simulink model "cruise_control_sim"  (R2013a)
settings: Solver=ode1  StartTime=0.0  StopTime=50  FixedStep=0.1  RelTol=1e-3
PreLoadFcn:
  | load('cruise_control_sim.mat')
undefined symbols (not defined in the file): EngineRPM, EngineTRQ, FinalRatio, GearRatio, Kdrag, Ki, Kp, Mass, sigbuilder_block, WheelRadius
libraries: simulink x1
settings Model: Creator=luca  LastModifiedBy=luca

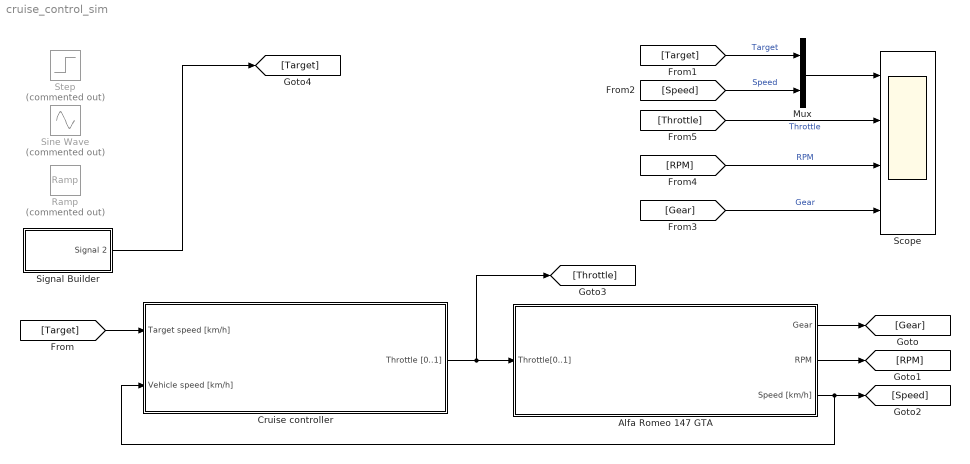
== system cruise_control_sim ==
  Alfa Romeo 147 GTA : Subsystem
  Cruise controller : Subsystem
  Mux : Mux  Inputs=2
  Ramp : simulink/Sources/Ramp  Commented=on  slope=6  start=0  X0=0
  Scope : Scope  NumInputPorts=4
      settings: ShowLegends=on  YMin=-5~-5~-5~-5  YMax=5~5~5~5
  Signal Builder : Subsystem  Tag=STV Subsys  LoadFcn=sigbuilder_block('load');  StartFcn=sigbuilder_block('start');  StopFcn=sigbuilder_block('stop');  ClipboardFcn=sigbuilder_block('clipboard');  mask(Sigbuilder block){}
      mask help: Simulink:masks:SigbuilderBlock_MD
      mask init:
      | if ~strcmp(get_param(bdroot(gcbh),'SimulationStatus'),'stopped') tuvar = sigbuilder_block('maskInit'); end
      settings: CopyFcn=sigbuilder_block('copy');  DeleteFcn=sigbuilder_block('delete');  ModelCloseFcn=sigbuilder_block('modelClose');  PreSaveFcn=sigbuilder_block('preSave');  PauseFcn=sigbuilder_block('pause');  ContinueFcn=sigbuilder_block('continue');  NameChangeFcn=sigbuilder_block('namechange');  OpenFcn=sigbuilder_block('open',[0 25.6 819.2 554.4 ]);  CloseFcn=sigbuilder_block('close');
      mask Display: plot(0, 0, 100, 100,[2, 2, 32, 32, 2], [68, 8, 8, 68, 68],[32, 2], [38, 38], [32, 19, 2],[53, 60, 44], [32, 17, 17, 2],[16, 16, 31, 31]);txt = getActiveGroup(gcbh);text(2, 100, txt,'verticalAlignment', 'top');
  Sine Wave : Sin  Commented=on  Amplitude=20  Bias=100  Frequency=0.2  SampleTime=0
  Step : Step  Commented=on  After=100  SampleTime=0
  wires:
  Cruise controller/1(Throttle [0..1]) -> Alfa Romeo 147 GTA/1(Throttle[0..1]), [Throttle]
  Alfa Romeo 147 GTA/3(Speed [km/h]) -> [Speed], Cruise controller/2(Vehicle speed [km/h])
  [Target] -> Cruise controller/1(Target speed [km/h])
  Alfa Romeo 147 GTA/1(Gear) -> [Gear]
  Alfa Romeo 147 GTA/2(RPM) -> [RPM]
  [Gear] -> Scope/4  "Gear"
  [RPM] -> Scope/3  "RPM"
  [Throttle] -> Scope/2  "Throttle"
  [Target] -> Mux/1  "Target"
  [Speed] -> Mux/2  "Speed"
  Mux/1 -> Scope/1
  Signal Builder/1(Signal 2) -> [Target]

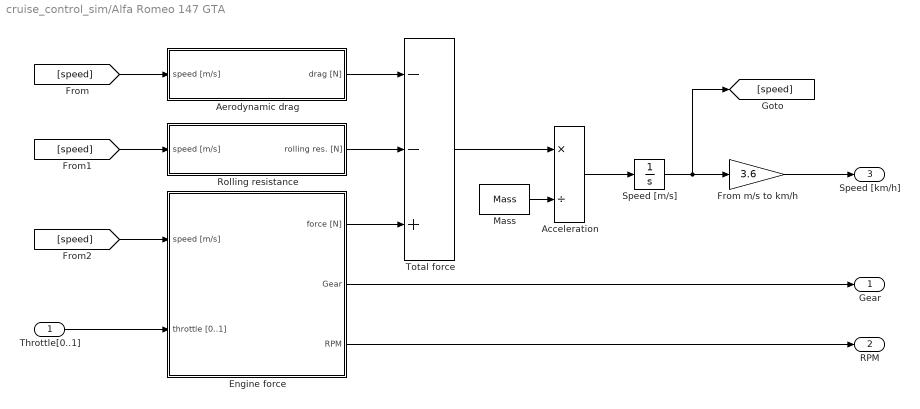
== system cruise_control_sim/Alfa Romeo 147 GTA ==
  Throttle[0..1] : Inport
  Acceleration : Product  Inputs=*/
  Aerodynamic drag : Subsystem
  Engine force : Subsystem
  From m/s to km/h : Gain  Gain=3.6
  Mass : Constant  Value=Mass
  Rolling resistance : Subsystem
  Speed [m/s] : Integrator
  Total force : Sum  Inputs=--+
  Gear : Outport
  RPM : Outport  Port=2
  Speed [km/h] : Outport  Port=3
  wires:
  Engine force/1(force [N]) -> Total force/3
  Rolling resistance/1(rolling res. [N]) -> Total force/2
  Aerodynamic drag/1(drag [N]) -> Total force/1
  Total force/1 -> Acceleration/1
  Mass/1 -> Acceleration/2
  Acceleration/1 -> Speed [m/s]/1
  Speed [m/s]/1 -> [speed], From m/s to km/h/1
  From m/s to km/h/1 -> Speed [km/h]/1
  [speed] -> Aerodynamic drag/1(speed [m/s])
  [speed] -> Rolling resistance/1(speed [m/s])
  Throttle[0..1]/1 -> Engine force/2(throttle [0..1])
  [speed] -> Engine force/1(speed [m/s])
  Engine force/2(Gear) -> Gear/1
  Engine force/3(RPM) -> RPM/1

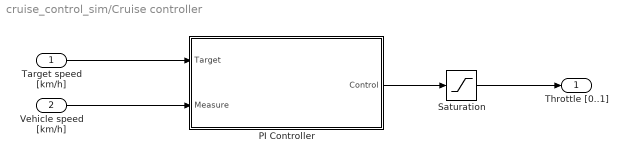
== system cruise_control_sim/Cruise controller ==
  Target speed [km/h] : Inport
  Vehicle speed [km/h] : Inport  Port=2
  PI Controller : Subsystem
  Saturation : Saturate  UpperLimit=1  LowerLimit=0
  Throttle [0..1] : Outport
  wires:
  Vehicle speed [km/h]/1 -> PI Controller/2(Measure)
  PI Controller/1(Control) -> Saturation/1
  Saturation/1 -> Throttle [0..1]/1
  Target speed [km/h]/1 -> PI Controller/1(Target)

== system cruise_control_sim/Signal Builder ==
  Demux : Demux  Tag=STV Demux  Outputs=1
  FromWs : FromWorkspace  Tag=STV FromWs  VariableName=tuvar  SampleTime=0
      SigBuilderData=|
      | common.afterFinalStr = 'Extrapolate'
      | common.sampleTime = 0
      | dataSet.timeRange = [0 50]
      | dataSet.name = 'Group 1'
      | sbobj.Groups.Name = 'Group 1'
      | sbobj.Groups.Signals.Name = 'Signal 2'
      | sbobj.Groups.Signals.XData = [0 5 5 10 10 20 20 30 30 40 40 50]
      | sbobj.Groups.Signals.YData = [30 30 50 50 80 80 100 100 120 120 140 140]
      | sbobj.Groups.TimeRange = [0 50]
  Signal 2 : Outport  Tag=STV Outport
  wires:
  FromWs/1 -> Demux/1
  Demux/1 -> Signal 2/1

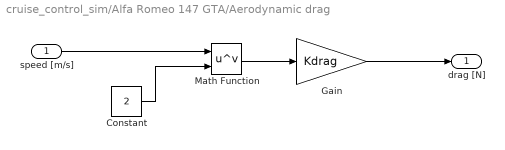
== system cruise_control_sim/Alfa Romeo 147 GTA/Aerodynamic drag ==
  speed [m/s] : Inport
  Constant : Constant  Value=2
  Gain : Gain  Gain=Kdrag
  Math Function : Math  Operator=pow  SaturateOnIntegerOverflow=on
  drag [N] : Outport
  wires:
  speed [m/s]/1 -> Math Function/1
  Constant/1 -> Math Function/2
  Math Function/1 -> Gain/1
  Gain/1 -> drag [N]/1

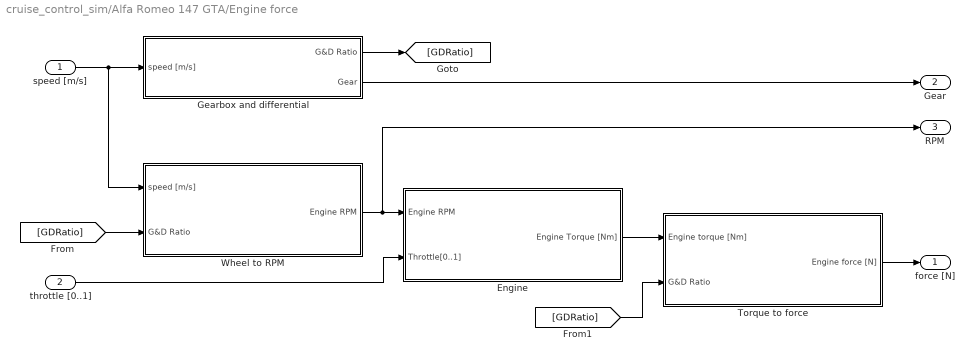
== system cruise_control_sim/Alfa Romeo 147 GTA/Engine force ==
  speed [m/s] : Inport
  throttle [0..1] : Inport  Port=2
  Engine : Subsystem
  Gearbox and differential : Subsystem
  Torque to force : Subsystem
  Wheel to RPM : Subsystem
  force [N] : Outport
  Gear : Outport  Port=2
  RPM : Outport  Port=3
  wires:
  Wheel to RPM/1(Engine RPM) -> RPM/1, Engine/1(Engine RPM)
  throttle [0..1]/1 -> Engine/2(Throttle[0..1])
  speed [m/s]/1 -> Gearbox and differential/1(speed [m/s]), Wheel to RPM/1(speed [m/s])
  Engine/1(Engine Torque [Nm]) -> Torque to force/1(Engine torque [Nm])
  Torque to force/1(Engine force [N]) -> force [N]/1
  Gearbox and differential/1(G&D Ratio) -> [GDRatio]
  [GDRatio] -> Wheel to RPM/2(G&D Ratio)
  [GDRatio] -> Torque to force/2(G&D Ratio)
  Gearbox and differential/2(Gear) -> Gear/1

== system cruise_control_sim/Alfa Romeo 147 GTA/Rolling resistance ==
  speed [m/s] : Inport
  Gain : Gain  Gain=30*Kdrag
  rolling res. [N] : Outport
  wires:
  speed [m/s]/1 -> Gain/1
  Gain/1 -> rolling res. [N]/1

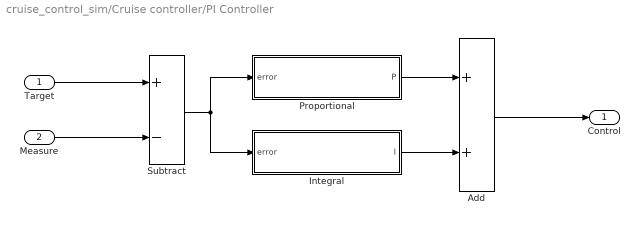
== system cruise_control_sim/Cruise controller/PI Controller ==
  Target : Inport
  Measure : Inport  Port=2
  Add : Sum
  Integral : Subsystem
  Proportional : Subsystem
  Subtract : Sum  Inputs=+-
  Control : Outport
  wires:
  Subtract/1 -> Integral/1(error), Proportional/1(error)
  Target/1 -> Subtract/1
  Measure/1 -> Subtract/2
  Integral/1(I) -> Add/2
  Proportional/1(P) -> Add/1
  Add/1 -> Control/1

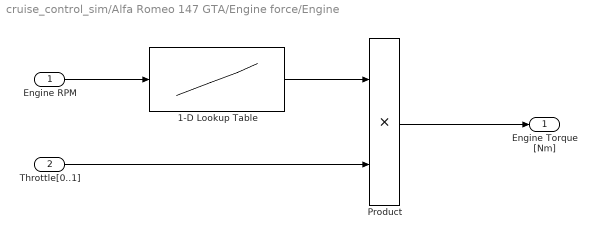
== system cruise_control_sim/Alfa Romeo 147 GTA/Engine force/Engine ==
  Engine RPM : Inport
  Throttle[0..1] : Inport  Port=2
  1-D Lookup Table : Lookup_n-D  NumberOfTableDimensions=1  BreakpointsForDimension1=EngineRPM  Table=EngineTRQ  InterpMethod=Cubic spline  RndMeth=Simplest  InputSameDT=on
  Product : Product
  Engine Torque [Nm] : Outport
  wires:
  Engine RPM/1 -> 1-D Lookup Table/1
  Throttle[0..1]/1 -> Product/2
  1-D Lookup Table/1 -> Product/1
  Product/1 -> Engine Torque [Nm]/1

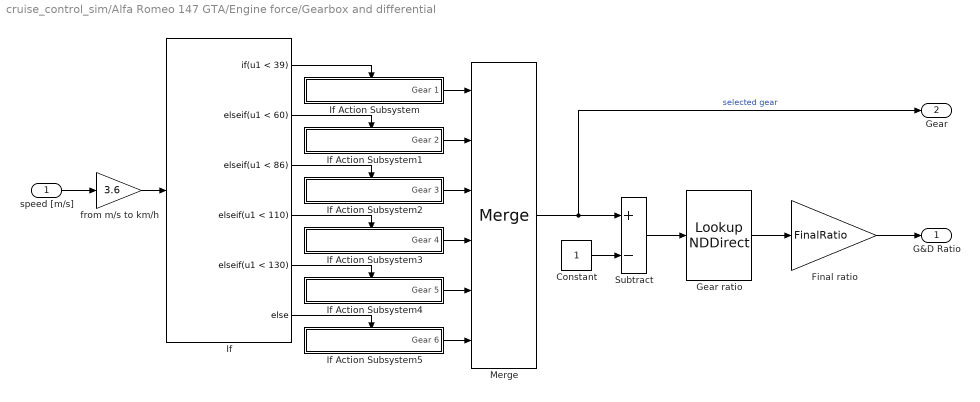
== system cruise_control_sim/Alfa Romeo 147 GTA/Engine force/Gearbox and differential ==
  speed [m/s] : Inport
  Constant : Constant
  Final ratio : Gain  Gain=FinalRatio
  Gear ratio : LookupNDDirect  NumberOfTableDimensions=1  Table=GearRatio
  If : If  IfExpression=u1 < 39  ElseIfExpressions=u1 < 60, u1 < 86, u1 < 110, u1 < 130
  If Action Subsystem : Subsystem  TreatAsAtomicUnit=on
  If Action Subsystem1 : Subsystem  TreatAsAtomicUnit=on
  If Action Subsystem2 : Subsystem  TreatAsAtomicUnit=on
  If Action Subsystem3 : Subsystem  TreatAsAtomicUnit=on
  If Action Subsystem4 : Subsystem  TreatAsAtomicUnit=on
  If Action Subsystem5 : Subsystem  TreatAsAtomicUnit=on
  Merge : Merge  Inputs=6
  Subtract : Sum  Inputs=+-
  from m/s to km/h : Gain  Gain=3.6
  G&D Ratio : Outport
  Gear : Outport  Port=2
  wires:
  speed [m/s]/1 -> from m/s to km/h/1
  from m/s to km/h/1 -> If/1
  If/1 -> If Action Subsystem/Action
  If/2 -> If Action Subsystem1/Action
  If/3 -> If Action Subsystem2/Action
  If/4 -> If Action Subsystem3/Action
  If/5 -> If Action Subsystem4/Action
  If/6 -> If Action Subsystem5/Action
  If Action Subsystem/1(Gear 1) -> Merge/1
  If Action Subsystem1/1(Gear 2) -> Merge/2
  If Action Subsystem2/1(Gear 3) -> Merge/3
  If Action Subsystem3/1(Gear 4) -> Merge/4
  If Action Subsystem4/1(Gear 5) -> Merge/5
  If Action Subsystem5/1(Gear 6) -> Merge/6
  Gear ratio/1 -> Final ratio/1
  Final ratio/1 -> G&D Ratio/1
  Merge/1 -> Gear/1, Subtract/1  "selected gear"
  Subtract/1 -> Gear ratio/1
  Constant/1 -> Subtract/2

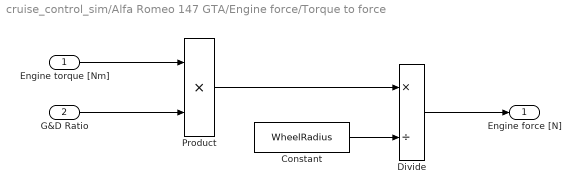
== system cruise_control_sim/Alfa Romeo 147 GTA/Engine force/Torque to force ==
  Engine torque [Nm] : Inport
  G&D Ratio : Inport  Port=2
  Constant : Constant  Value=WheelRadius
  Divide : Product  Inputs=*/
  Product : Product
  Engine force [N] : Outport
  wires:
  Engine torque [Nm]/1 -> Product/1
  G&D Ratio/1 -> Product/2
  Product/1 -> Divide/1
  Constant/1 -> Divide/2
  Divide/1 -> Engine force [N]/1

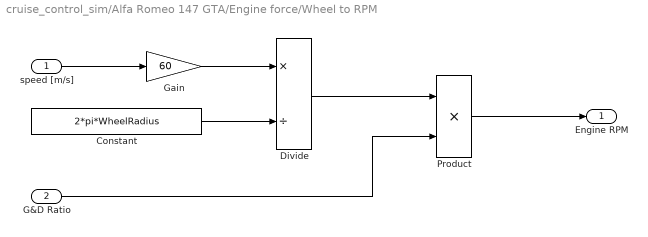
== system cruise_control_sim/Alfa Romeo 147 GTA/Engine force/Wheel to RPM ==
  speed [m/s] : Inport
  G&D Ratio : Inport  Port=2
  Constant : Constant  Value=2*pi*WheelRadius
  Divide : Product  Inputs=*/
  Gain : Gain  Gain=60
  Product : Product
  Engine RPM : Outport
  wires:
  speed [m/s]/1 -> Gain/1
  Gain/1 -> Divide/1
  Constant/1 -> Divide/2
  Divide/1 -> Product/1
  G&D Ratio/1 -> Product/2
  Product/1 -> Engine RPM/1

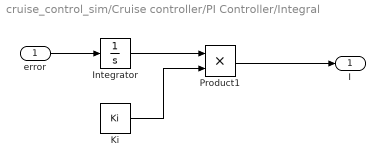
== system cruise_control_sim/Cruise controller/PI Controller/Integral ==
  error : Inport
  Integrator : Integrator
  Ki : Constant  Value=Ki
  Product1 : Product
  I : Outport
  wires:
  Ki/1 -> Product1/2
  Integrator/1 -> Product1/1
  Product1/1 -> I/1
  error/1 -> Integrator/1

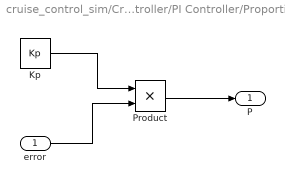
== system cruise_control_sim/Cruise controller/PI Controller/Proportional ==
  error : Inport
  Kp : Constant  Value=Kp
  Product : Product
  P : Outport
  wires:
  Kp/1 -> Product/1
  Product/1 -> P/1
  error/1 -> Product/2

== system cruise_control_sim/Alfa Romeo 147 GTA/Engine force/Gearbox and differential/If Action Subsystem ==
  Action Port : ActionPort  ActionType=then
  Constant : Constant
  Gear 1 : Outport  InitialOutput=1
  wires:
  Constant/1 -> Gear 1/1

== system cruise_control_sim/Alfa Romeo 147 GTA/Engine force/Gearbox and differential/If Action Subsystem1 ==
  Action Port : ActionPort  ActionType=elseif
  Constant : Constant  Value=2
  Gear 2 : Outport  InitialOutput=2
  wires:
  Constant/1 -> Gear 2/1

== system cruise_control_sim/Alfa Romeo 147 GTA/Engine force/Gearbox and differential/If Action Subsystem2 ==
  Action Port : ActionPort  ActionType=elseif
  Constant : Constant  Value=3
  Gear 3 : Outport  InitialOutput=3
  wires:
  Constant/1 -> Gear 3/1

== system cruise_control_sim/Alfa Romeo 147 GTA/Engine force/Gearbox and differential/If Action Subsystem3 ==
  Action Port : ActionPort  ActionType=elseif
  Constant : Constant  Value=4
  Gear 4 : Outport  InitialOutput=4
  wires:
  Constant/1 -> Gear 4/1

== system cruise_control_sim/Alfa Romeo 147 GTA/Engine force/Gearbox and differential/If Action Subsystem4 ==
  Action Port : ActionPort  ActionType=elseif
  Constant : Constant  Value=5
  Gear 5 : Outport  InitialOutput=5
  wires:
  Constant/1 -> Gear 5/1

== system cruise_control_sim/Alfa Romeo 147 GTA/Engine force/Gearbox and differential/If Action Subsystem5 ==
  Action Port : ActionPort  ActionType=else
  Constant : Constant  Value=6
  Gear 6 : Outport  InitialOutput=6
  wires:
  Constant/1 -> Gear 6/1
